simulink model "zad2"  (R2024a)
settings: Solver=VariableStepAuto  StartTime=0.0  StopTime=10.0  RelTol=1e-3
undefined symbols (not defined in the file): A, alfa, B, c, F, F4, k, m, M
settings Model: Creator=adasf  LastModifiedBy=adasf

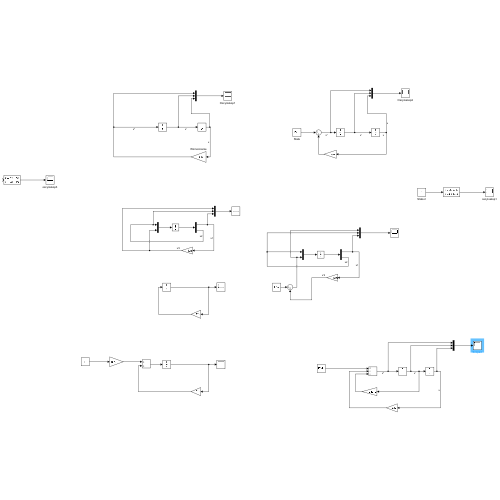
[thumbnail: Simulink's stored preview of the top-level diagram]
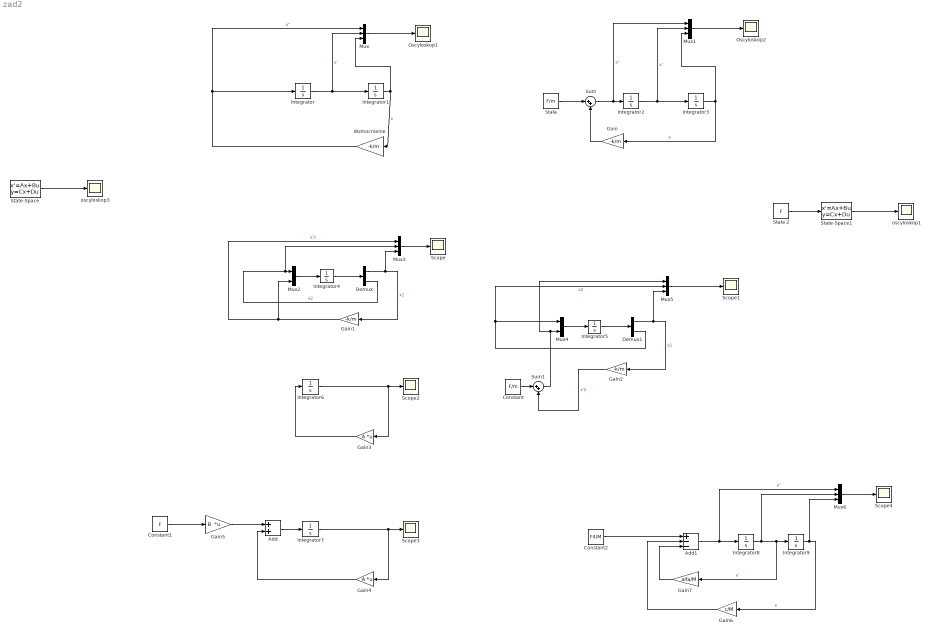
== system zad2 ==
  Add : Sum
  Add1 : Sum  Inputs=+--
  Constant : Constant  Value=F/m
  Constant1 : Constant  Value=F
  Constant2 : Constant  Value=F4/M
  Demux : Demux  Outputs=2
  Demux1 : Demux  Outputs=2
  Gain : Gain  Gain=-k/m
  Gain1 : Gain  Gain=-k/m
  Gain2 : Gain  Gain=-k/m
  Gain3 : Gain  Gain=A  Multiplication=Matrix(K*u)
  Gain4 : Gain  Gain=A  Multiplication=Matrix(K*u)
  Gain5 : Gain  Gain=B  Multiplication=Matrix(K*u)
  Gain6 : Gain  Gain=c/M
  Gain7 : Gain  Gain=alfa/M
  Integrator{,2,8..9} (4 alike) : Integrator
  Integrator1 : Integrator  InitialCondition=0.1
  Integrator3 : Integrator  InitialCondition=0.1
  Integrator{4..7} (4 alike) : Integrator  InitialCondition=[0.1; 0]
  Mux{,1,3,5..6} (5 alike) : Mux  Inputs=3
  Mux2 : Mux  Inputs=2
  Mux4 : Mux  Inputs=2
  Oscyloskop1 : Scope
  Oscyloskop2 : Scope
  Scope{,1..4} (5 alike) : Scope
  State-Space : StateSpace  A=[0 1 ; -k/m 0]  B=[0 ; 0]  C=[1 0 ;0 1 ]  D=[0 ;0]  InitialCondition=[0.1 ; 0]
  State-Space1 : StateSpace  A=[0 1 ; -k/m 0]  B=[0 ; 1/m]  C=[1 0 ;0 1 ]  D=[0 ;0]  InitialCondition=[0.1 ; 0]
  Stała : Constant  Value=F/m
  Stała 2 : Constant  Value=F
  Sum : Sum  Inputs=|++
  Sum1 : Sum  Inputs=|++
  Wzmocnienie : Gain  Gain=-k/m
  oscyloskop1 : Scope
  oscyloskop3 : Scope
  wires:
  Integrator/1 -> Mux/2, Integrator1/1  "x'"
  Integrator1/1 -> Mux/3, Wzmocnienie/1  "x"
  Wzmocnienie/1 -> Integrator/1, Mux/1  "x\""
  Mux/1 -> Oscyloskop1/1
  Stała/1 -> Sum/1
  Gain/1 -> Sum/2
  Integrator3/1 -> Gain/1, Mux1/3  "x"
  Integrator2/1 -> Mux1/2, Integrator3/1  "x'"
  Mux1/1 -> Oscyloskop2/1
  Sum/1 -> Mux1/1, Integrator2/1  "x\""
  State-Space/1 -> oscyloskop3/1
  State-Space1/1 -> oscyloskop1/1
  Stała 2/1 -> State-Space1/1
  Mux2/1 -> Integrator4/1
  Integrator4/1 -> Demux/1
  Demux/1 -> Mux3/3, Gain1/1  "x1"
  Mux3/1 -> Scope/1
  Gain1/1 -> Mux3/1, Mux2/2  "x'2"
  Demux/2 -> Mux3/2, Mux2/1  "x2"
  Mux5/1 -> Scope1/1
  Integrator5/1 -> Demux1/1
  Mux4/1 -> Integrator5/1
  Demux1/1 -> Mux5/3, Gain2/1  "x1"
  Gain2/1 -> Sum1/2  "x'2"
  Demux1/2 -> Mux4/1, Mux5/2  "x2"
  Constant/1 -> Sum1/1
  Sum1/1 -> Mux5/1, Mux4/2
  Integrator6/1 -> Gain3/1, Scope2/1
  Gain3/1 -> Integrator6/1
  Integrator7/1 -> Gain4/1, Scope3/1
  Gain5/1 -> Add/1
  Gain4/1 -> Add/2
  Add/1 -> Integrator7/1
  Constant1/1 -> Gain5/1
  Constant2/1 -> Add1/1
  Add1/1 -> Mux6/1, Integrator8/1  "x\""
  Integrator8/1 -> Mux6/2, Gain7/1, Integrator9/1  "x'"
  Integrator9/1 -> Mux6/3, Gain6/1  "x"
  Gain7/1 -> Add1/3
  Gain6/1 -> Add1/2
  Mux6/1 -> Scope4/1
